simulink model "temp_sim"  (R2021a)
settings: Solver=FixedStepAuto  StartTime=0.0  StopTime=10.0  FixedStep=1e-3  RelTol=1e-3
values from neighbouring files (symbols this model uses):
  Ku = 5    [temp_scri.m]
  tau = 5    [temp_scri.m]
settings Model: Creator=AHMED  LastModifiedBy=AHMED
settings OptimizationCC: DefaultParameterBehavior=Inlined  UseDivisionForNetSlopeComputation=on  GainParamInheritBuiltInType=on  UseFloatMulNetSlope=on  InlineInvariantSignals=on  PassReuseOutputArgsAs=Individual arguments  ZeroExternalMemoryAtStartup=off  ZeroInternalMemoryAtStartup=off  NoFixptDivByZeroProtection=on  EfficientFloat2IntCast=on  LifeSpan=1  OptimizeBlockOrder=speed  DifferentSizesBufferReuse=on  EfficientTunableParamExpr=on
settings DebuggingCC: ParameterTunabilityLossMsg=error
settings HardwareCC: ProdBitPerInt=16  ProdBitPerPointer=8  ProdBitPerSizeT=24  ProdBitPerPtrDiffT=24  ProdLargestAtomicFloat=None  ProdWordSize=8  ProdLongLongMode=on  ProdHWDeviceType=Microchip->PIC18
settings SFSimCC: MATLABDynamicMemAlloc=off
settings RTWCC: SystemTargetFile=ert.tlc  TemplateMakefile=ert_default_tmf
settings CodeAppCC: ForceParamTrailComments=on  IgnoreCustomStorageClasses=off  OperatorAnnotations=on  SimulinkDataObjDesc=on  SFDataObjDesc=on  CustomSymbolStrGlobalVar=rt$N$M  CustomSymbolStrType=$N$M  CustomSymbolStrFcn=$N$M$F  CustomSymbolStrMacro=$N$M  InsertBlockDesc=on
settings ERTTargetCC: TargetLangStandard=C99 (ISO)  GenerateSampleERTMain=on  IncludeMdlTerminateFcn=off  CombineSignalStateStructs=on  SupportComplex=off  SupportContinuousTime=on  InlinedParameterPlacement=NonHierarchical  ERTCustomFileTemplate=example_file_process.tlc  ERTFilePackagingFormat=CompactWithDataFile

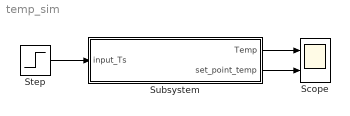
== system temp_sim ==
  Scope : Scope  NumInputPorts=2
  Step : Step  After=10  SampleTime=0
  Subsystem : Subsystem
  wires:
  Step/1 -> Subsystem/1(input_Ts)
  Subsystem/1(Temp) -> Scope/1
  Subsystem/2(set_point_temp) -> Scope/2

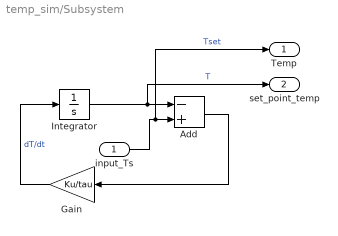
== system temp_sim/Subsystem ==
  input_Ts : Inport
  Add : Sum  Inputs=-+
  Gain : Gain  Gain=Ku/tau
  Integrator : Integrator
  Temp : Outport
  set_point_temp : Outport  Port=2
  wires:
  Integrator/1 -> set_point_temp/1, Add/1  "T"
  Add/1 -> Gain/1
  input_Ts/1 -> Temp/1, Add/2  "Tset"
  Gain/1 -> Integrator/1  "dT/dt"
